simulink model "acquisition"  (Simulink 8.1)
settings: Solver=ode45  StartTime=0.0  StopTime=10.0  RelTol=1e-3
undefined symbols (not defined in the file or in its folder): magnitude
libraries: dspxfrm3 x4, powerlib_extras x2, commsynccomp2 x2, dspsrcs4 x2
settings Model: Creator=SISA  LastModifiedBy=cfuiugt6s4pkhdrji0

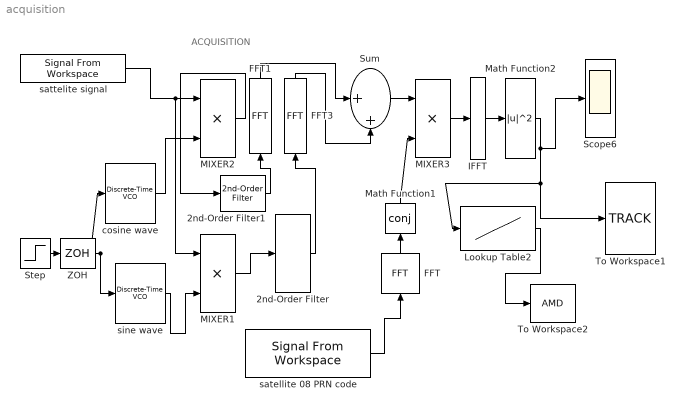
== system acquisition ==
  note: ACQUISITION
  2nd-Order Filter : powerlib_extras/Control  Blocks/2nd-Order Filter  FilterType=Lowpass  Fo=50  Zeta=0.707  Initialize=off  Vac_Init=[1 45 60]  Vdc_Init=-0.5  PlotResponse=off  param1=[1 500 1]
  2nd-Order Filter1 : powerlib_extras/Control  Blocks/2nd-Order Filter  FilterType=Lowpass  Fo=50  Zeta=0.707  Initialize=off  Vac_Init=[1 45 60]  Vdc_Init=-0.5  PlotResponse=off  param1=[1 500 1]
  FFT : dspxfrm3/FFT  CompMethod=Table lookup  TableOpt=NEW  TableOptActive=Speed  BitRevOrder=off  InheritFFTLength=on  FFTLength=64  RowConvenienceOn=on  FFTImplementation=Auto  SkipNorm=off  firstCoeffDataTypeStr=Inherit: Same word length as input  firstCoeffLastDataTypeStr=Inherit: Same word length as input  outputMin=[]  outputMax=[]  roundingMode=Floor  overflowMode=off
  FFT1 : dspxfrm3/FFT  CompMethod=Table lookup  TableOpt=NEW  TableOptActive=Speed  BitRevOrder=off  InheritFFTLength=on  FFTLength=64  RowConvenienceOn=on  FFTImplementation=Auto  SkipNorm=off  firstCoeffDataTypeStr=Inherit: Same word length as input  firstCoeffLastDataTypeStr=Inherit: Same word length as input  outputMin=[]  outputMax=[]  roundingMode=Floor  overflowMode=off
  FFT3 : dspxfrm3/FFT  CompMethod=Table lookup  TableOpt=NEW  TableOptActive=Speed  BitRevOrder=off  InheritFFTLength=on  FFTLength=64  RowConvenienceOn=on  FFTImplementation=Auto  SkipNorm=off  firstCoeffDataTypeStr=Inherit: Same word length as input  firstCoeffLastDataTypeStr=Inherit: Same word length as input  outputMin=[]  outputMax=[]  roundingMode=Floor  overflowMode=off
  IFFT : dspxfrm3/IFFT  CompMethod=Table lookup  TableOpt=NEW  TableOptActive=Speed  BitRevOrder=off  cs_in=off  SkipNorm=on  InheritFFTLength=on  FFTLength=64  mode=Complex  outSamplingMode=Sample based  RowConvenienceOn=on  FFTImplementation=Auto  firstCoeffDataTypeStr=Inherit: Same word length as input  firstCoeffLastDataTypeStr=Inherit: Same word length as input  outputMin=[]  outputMax=[]  roundingMode=Floor  overflowMode=off
  Lookup Table2 : Lookup  InputValues=[0,1]  Table=[0,1]  LookUpMeth=Use Input Above
  MIXER1 : Product  RndMeth=Zero
  MIXER2 : Product  RndMeth=Zero
  MIXER3 : Product  RndMeth=Zero
  Math Function1 : Math  Operator=conj  OutputSignalType=complex  SaturateOnIntegerOverflow=on
  Math Function2 : Math  Operator=magnitude^2  OutputSignalType=real  SaturateOnIntegerOverflow=on
  Scope6 : Scope
  Step : Step  SampleTime=0
  Sum : Sum  Inputs=|++
  To Workspace1 : ToWorkspace  VariableName=TRACK  SampleTime=-1
      settings: MaxDataPoints=1023000
  To Workspace2 : ToWorkspace  VariableName=AMD  SampleTime=-1
      settings: MaxDataPoints=1023000
  ZOH : ZeroOrderHold
  cosine wave : commsynccomp2/Discrete-Time VCO  Ac=3  Fc=7000000  Kc=1  Ph=0  ts=0.01
  satellite 08 PRN code : dspsrcs4/Signal From Workspace  X=PN08  Ts=1  nsamps=1  OutputAfterFinalValue=Setting to zero  ignoreOrWarnInputAndFrameLengths=off
  sattelite signal : dspsrcs4/Signal From Workspace  X=COM1  Ts=1  nsamps=1  OutputAfterFinalValue=Setting to zero  ignoreOrWarnInputAndFrameLengths=off
  sine wave : commsynccomp2/Discrete-Time VCO  Ac=3  Fc=7000000  Kc=1  Ph=-pi/2  ts=0.01
  wires:
  sattelite signal/1 -> MIXER2/1, MIXER1/1
  Step/1 -> ZOH/1
  ZOH/1 -> cosine wave/1, sine wave/1
  cosine wave/1 -> MIXER2/2
  sine wave/1 -> MIXER1/2
  Sum/1 -> MIXER3/1
  FFT1/1 -> Sum/1
  FFT3/1 -> Sum/2
  Math Function1/1 -> MIXER3/2
  FFT/1 -> Math Function1/1
  satellite 08 PRN code/1 -> FFT/1
  Math Function2/1 -> Scope6/1, To Workspace1/1, Lookup Table2/1
  IFFT/1 -> Math Function2/1
  MIXER3/1 -> IFFT/1
  Lookup Table2/1 -> To Workspace2/1
  MIXER2/1 -> 2nd-Order Filter1/1
  2nd-Order Filter1/1 -> FFT1/1
  2nd-Order Filter/1 -> FFT3/1
  MIXER1/1 -> 2nd-Order Filter/1
